simulink model "Unsymmetrical"  (R2021a)
settings: Solver=VariableStepAuto  StartTime=0.0  StopTime=0.5  RelTol=1e-3
undefined symbols (not defined in the file): D11, Delta
libraries: spsCurrentMeasurementLib x3, spsThreePhaseSeriesRLCLoadLib x2, spsExcitationSystemLib x1, spsHydraulicTurbineandGovernorLib x1, spsThreePhaseSourceLib x1, spsSynchronousMachinepuFundamentalLib x1, spsThreePhasePISectionLineLib x1, spsThreePhaseTransformerTwoWindingsLib x1, spsThreePhaseVIMeasurementLib x1, spsThreePhaseFaultLib x1, spspowerguiLib x1
settings Model: Creator=saika  LastModifiedBy=saika

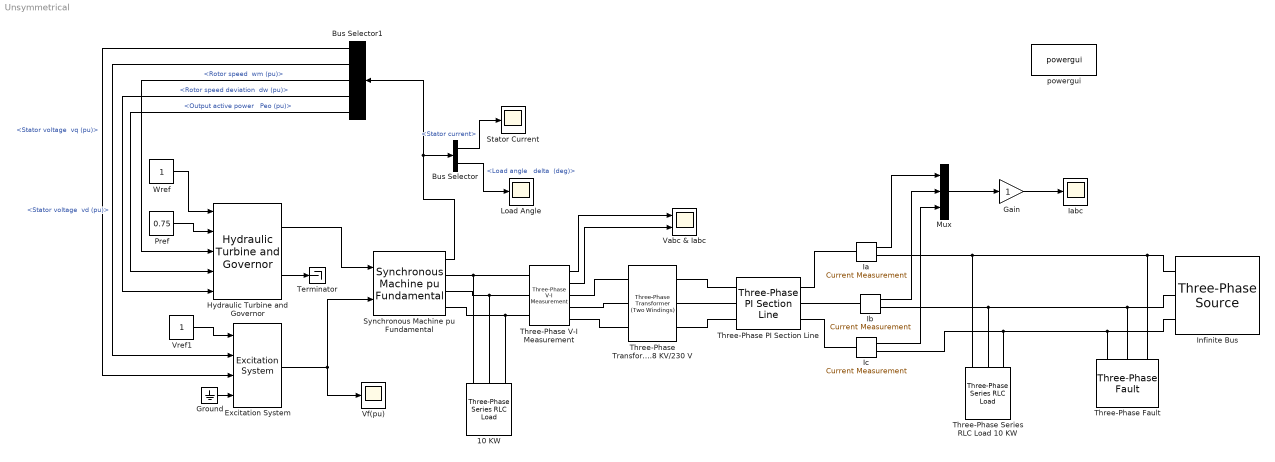
== system Unsymmetrical ==
  10 KW : spsThreePhaseSeriesRLCLoadLib/Three-Phase Series RLC Load  LConnTagsString=A|B|C  Configuration=Y (grounded)  NominalVoltage=13.8e3  Vabc=[1e3 1e3 1e3]  Vabcp=[1e3 1e3 1e3]  NominalFrequency=50  UnbalancedPower=off  ActivePower=10e3  InductivePower=0  CapacitivePower=0  Pabc=[10e3 9e3 11e3]  QLabc=[100 90 110]  QCabc=[100 90 110]  Pabcp=[10e3 9e3 11e3]  QLabcp=[100 90 110]  QCabcp=[100 90 110]  Measurements=None  LoadType=constant Z
  Bus Selector : BusSelector  OutputSignals="Stator current,Load angle   delta  (deg)"
  Bus Selector1 : BusSelector  OutputSignals="dq0 components.Stator voltage  vq (pu),dq0 components.Stator voltage  vd (pu),Mechanical.Rotor speed  wm (pu),Mechanical.Rotor speed deviation  dw (pu),Output active power   Peo (pu)"
  Excitation System : spsExcitationSystemLib/Excitation System  tr=20e-3  reg=[ 300, 0.001 ]  exc=[ 1, 0 ]  tgr=[ 0, 0 ]  damp=[ 0.001, 0.1 ]  sat=[ 0, 0 ]  lim=[ -11.5, 11.5, 0 ]  v0="[1.0  1.28]"
      settings: SourceProductBaseCode=PS
  Gain : Gain
  Ground : Ground
  Hydraulic Turbine and Governor : spsHydraulicTurbineandGovernorLib/Hydraulic Turbine and Governor  sm="[ 10/3  0.07 ]"  gate="[  0.01  0.97518  -0.1  0.1 ]"  reg="[  0.05  1.163  0.105  0  0.01  ]"  hyd="[  0  2.67  ]"  dref=0  po=0.7516
      settings: SourceProductBaseCode=PS
  Ia : spsCurrentMeasurementLib/Current Measurement  PhasorSimulation=off  OutputType=Complex  PSBequivalent=0
  Iabc : Scope
  Ib : spsCurrentMeasurementLib/Current Measurement  PhasorSimulation=off  OutputType=Complex  PSBequivalent=0
  Ic : spsCurrentMeasurementLib/Current Measurement  PhasorSimulation=off  OutputType=Complex  PSBequivalent=0
  Infinite Bus : spsThreePhaseSourceLib/Three-Phase Source  InternalConnection=Yg  VoltagePhases=off  Voltage=230e3  PhaseAngle=0  Voltage_phases=[25e3 25e3 25e3]/sqrt(3)  PhaseAngles_phases=[0 -120 +120]  Frequency=50  NonIdealSource=on  SpecifyImpedance=off  Resistance=0.8929  Inductance=16.58e-3  ShortCircuitLevel=100e6  BaseVoltage=25e3  XRratio=7  BusType=swing  Pref=10e3  Qref=0  Prefabc=[10e3, 10e3, 10e3]  Qrefabc=[0, 0, 0]  Qmin=-inf  Qmax=inf
  Load Angle : Scope
  Mux : Mux  Inputs=3
  Pref : Constant  Value=0.75
  Stator Current : Scope
  Synchronous Machine pu Fundamental : spsSynchronousMachinepuFundamentalLib/Synchronous Machine pu Fundamental  PresetModel=No  MechanicalLoad=Mechanical power Pm  ShowDetailedParameters=on  RotorType=Salient-pole  Units=per unit fundamental parameters  MeasurementBus=off  NominalParameters="[ 200E6  13.8e3   50]"  Stator="[ 2.85E-03  0.114  1.19  0.36 ]"  Field="[ 5.79E-04  0.114]"  Dampers2=[0.0652, 0.5134, 0.0287, 0.2553, 7.765e-3, 0.9167 ]  Dampers1="[ 1.17E-02  0.182  1.97E-02  0.384 ]"  Mechanical=[ 3.7 0 20]  PolePairs=20  InitialConditions="[ 0  0  0  0  0  0  0  0  1 ]"  SetSaturation=off  Saturation=[0.6404,0.7127,0.8441,0.9214,0.9956,1.082,1.19,1.316,1.457;0.7,0.7698,0.8872,0.9466,0.9969,1.046,1.1,1.151,1.201]  LoadFlowParameters=[1,0,0,0,0]  TsPowergui=0  TsBlock=-1  IterativeModel=Trapezoidal non iterative  IterativeDiscreteModel=Trapezoidal non iterative  BusType=PV  Pref=0  Qref=0  Qmin=-inf  Qmax=inf  PLF=0  QLF=0
      settings: SourceProductBaseCode=PS
  Terminator : Terminator
  Three-Phase PI Section Line : spsThreePhasePISectionLineLib/Three-Phase PI Section Line  LConnTagsString=a|b|c  RConnTagsString=A|B|C  Length=100  Frequency=50  Resistances=[ 0.01273 0.3864]  Inductances="[ 0.9337e-3  4.1264e-3]"  Capacitances=[12.74e-9 7.751e-9]
  Three-Phase Series RLC Load 10 KW : spsThreePhaseSeriesRLCLoadLib/Three-Phase Series RLC Load  LConnTagsString=A|B|C  Configuration=Y (grounded)  NominalVoltage=1000  Vabc=[1e3 1e3 1e3]  Vabcp=[1e3 1e3 1e3]  NominalFrequency=50  UnbalancedPower=off  ActivePower=10e3  InductivePower=100  CapacitivePower=100  Pabc=[10e3 9e3 11e3]  QLabc=[100 90 110]  QCabc=[100 90 110]  Pabcp=[10e3 9e3 11e3]  QLabcp=[100 90 110]  QCabcp=[100 90 110]  Measurements=None  LoadType=constant Z
  Three-Phase Transformer 210 MVA,13.8 KV/230 V : spsThreePhaseTransformerTwoWindingsLib/Three-Phase Transformer (Two Windings)  Winding1Connection=Delta (D11)  Winding2Connection=Yg  CoreType=Three single-phase transformers  SetSaturation=off  Hysteresis=off  DataFile='hysteresis'  SetInitialFlux=off  Measurements=None  UNITS=pu  NominalPower=[ 210e6 , 50 ]  Winding1=[ 13.8e3 , 0.0027 , 0.08 ]  Winding2=[ 230e3 , 0.0027 , 0.08 ]  Rm=500.01  Lm=500  L0=0.5  Saturation=[ 0,0 ; 0.0024,1.2 ; 1.0,1.52 ]  InitialFluxes=[ 0.8 , -0.8 , 0.7 ]  BreakLoop=off  DiscreteSolver=Trapezoidal iterative  DataType=off  TransfoNumber=1
  Three-Phase V-I Measurement : spsThreePhaseVIMeasurementLib/Three-Phase V-I Measurement  VoltageMeasurement=phase-to-ground  SetLabelV=off  LabelV=Vabc  Vpu=off  VpuLL=off  CurrentMeasurement=yes  SetLabelI=off  LabelI=Iabc  Ipu=off  Pbase=100e6  Vbase=500e3  OutputType=Complex  PhasorSimulation=off  PSBequivalent=0
  Three-Phase Fault : spsThreePhaseFaultLib/Three-Phase Fault  InitialStates=0  FaultA=on  FaultB=on  FaultC=off  GroundFault=off  SwitchTimes=[0.2 0.3]  External=off  SwitchStatus=NaN  FaultResistance=1  GroundResistance=1  SnubberResistance=inf  SnubberCapacitance=inf  Measurements=None
  Vabc & Iabc : Scope  NumInputPorts=2
  Vf(pu) : Scope
  Vref1 : Constant
  Wref : Constant
  powergui : spspowerguiLib/powergui  Priority=1  SimulationMode=Discrete  SampleTime=50e-6  frequency=60  Iterations=50  frequencyindice=50  Pbase=100e6  ErrMax=1e-4  UnitsV=kV  UnitsW=MW  buscounter=0  FunctionMessages=off  echomessages=off  EnableUseOfTLC=off  CurrentSourceSwitches=off  DisableSnubberDevices=off  DisableRonSwitches=off  DisableVfSwitches=off  DisplayEquations=off  AutomaticDiscreteSolvers=off  SolverType=Backward Euler  Interpol=off  ExternalGateDelay=off  methode=off  Ts=100  x0status=blocks  SPID=on  SwTol=0  HookPort=off  NonlinearTolerance=1e-4  nMaxIteration=100  ContinueOnMaxIteration=off  RestoreLinks=warning  ResistiveCurrentMeasurement=off  Frange=[0:2:500]  Ylog=off  Xlog=on  ShowGrid=off  save=off  variable=ZData  structure=0  ZoomFFT=off  StartTime=0.0  cycles=1  DisplayStyle=1  fundamental=60  FreqAxis=off  MaxFrequency=1000  frequencyindicesteady=1  RmsSteady=1  display=off
  wires:
  Mux/1 -> Gain/1
  Bus Selector/1 -> Stator Current/1  "<Stator current>"
  Ic/1 -> Mux/3
  Synchronous Machine pu Fundamental/1 -> Bus Selector1/1, Bus Selector/1
  Gain/1 -> Iabc/1
  Bus Selector1/3 -> Hydraulic Turbine and Governor/3  "<Rotor speed  wm (pu)>"
  Ground/1 -> Excitation System/4
  Bus Selector1/2 -> Excitation System/2  "<Stator voltage  vd (pu)>"
  Ia/1 -> Mux/1
  Bus Selector1/5 -> Hydraulic Turbine and Governor/4  "<Output active power   Peo (pu)>"
  Vref1/1 -> Excitation System/1
  Wref/1 -> Hydraulic Turbine and Governor/1
  Bus Selector/2 -> Load Angle/1  "<Load angle   delta  (deg)>"
  Hydraulic Turbine and Governor/2 -> Terminator/1
  Three-Phase V-I Measurement/1 -> Vabc & Iabc/1
  Pref/1 -> Hydraulic Turbine and Governor/2
  Bus Selector1/1 -> Excitation System/3  "<Stator voltage  vq (pu)>"
  Ib/1 -> Mux/2
  Excitation System/1 -> Synchronous Machine pu Fundamental/2, Vf(pu)/1
  Three-Phase V-I Measurement/2 -> Vabc & Iabc/2
  Bus Selector1/4 -> Hydraulic Turbine and Governor/5  "<Rotor speed deviation  dw (pu)>"
  Hydraulic Turbine and Governor/1 -> Synchronous Machine pu Fundamental/1
  connections:
  Infinite Bus/RConn1 -- Ia/RConn1 -- Three-Phase Series RLC Load 10 KW/LConn1 -- Three-Phase Fault/LConn1
  Infinite Bus/RConn2 -- Ib/RConn1 -- Three-Phase Series RLC Load 10 KW/LConn2 -- Three-Phase Fault/LConn2
  10 KW/LConn1 -- Synchronous Machine pu Fundamental/RConn1 -- Three-Phase V-I Measurement/LConn1
  Three-Phase V-I Measurement/LConn2 -- Synchronous Machine pu Fundamental/RConn2 -- 10 KW/LConn2
  Three-Phase Series RLC Load 10 KW/LConn3 -- Ic/RConn1 -- Three-Phase Fault/LConn3 -- Infinite Bus/RConn3
  10 KW/LConn3 -- Synchronous Machine pu Fundamental/RConn3 -- Three-Phase V-I Measurement/LConn3
  Ib/LConn1 -- Three-Phase PI Section Line/RConn2
  Ic/LConn1 -- Three-Phase PI Section Line/RConn3
  Ia/LConn1 -- Three-Phase PI Section Line/RConn1
  Three-Phase Transformer 210 MVA,13.8 KV/230 V/LConn1 -- Three-Phase V-I Measurement/RConn1
  Three-Phase PI Section Line/LConn1 -- Three-Phase Transformer 210 MVA,13.8 KV/230 V/RConn1
  Three-Phase Transformer 210 MVA,13.8 KV/230 V/LConn2 -- Three-Phase V-I Measurement/RConn2
  Three-Phase V-I Measurement/RConn3 -- Three-Phase Transformer 210 MVA,13.8 KV/230 V/LConn3
  Three-Phase Transformer 210 MVA,13.8 KV/230 V/RConn2 -- Three-Phase PI Section Line/LConn2
  Three-Phase Transformer 210 MVA,13.8 KV/230 V/RConn3 -- Three-Phase PI Section Line/LConn3
